simulink model "test2"  (R2020b)
settings: Solver=FixedStepAuto  StartTime=0.0  StopTime=10.0  RelTol=1e-3
model workspace (MAT data in the model file):
  HDLVAXIMasterConfig = hdlverifier.internal.AXIMaster.ConfigParams
libraries: hdlsllib x38
(part 1 of 2)
settings Model: Creator=horse  LastModifiedBy=horse
settings OptimizationCC: BlockReduction=off  ConditionallyExecuteInputs=off  DefaultParameterBehavior=Inlined  OptimizeBlockIOStorage=off
settings HardwareCC: TargetBitPerPointer=64  TargetBitPerSizeT=64  TargetBitPerPtrDiffT=64  TargetLongLongMode=on  TargetIntDivRoundTo=Zero  TargetEndianess=LittleEndian  TargetWordSize=64  TargetHWDeviceType=Generic->Custom  ProdEqTarget=off
settings RTWCC: Description=SystemVerilog DPI Component Generator  SystemTargetFile=systemverilog_dpi_grt.tlc  TemplateMakefile=systemverilog_dpi_grt_default_tmf
settings CodeAppCC: MaxIdLength=256
settings DPIGRTTargetCC: TargetFcnLib=ansi_tfl_table_tmw.mat  GenFloatMathFcnCalls=NOT IN USE  TargetLangStandard=C89/C90 (ANSI)  CodeReplacementLibrary=None  UtilityFuncGeneration=Auto  MultiwordTypeDef=System defined  MultiwordLength=2048  DynamicStringBufferSize=256  GenerateFullHeader=on  InferredTypesCompatibility=off  GenerateSampleERTMain=off  GenerateTestInterfaces=off  ModelReferenceCompliant=on  ParMdlRefBuildCompliant=on  CompOptLevelCompliant=off  ConcurrentExecutionCompliant=off  IncludeMdlTerminateFcn=on  CombineOutputUpdateFcns=off  CombineSignalStateStructs=on  GroupInternalDataByFunction=off  SuppressErrorStatus=off  IncludeFileDelimiter=Auto  ERTCustomFileBanners=off  SupportAbsoluteTime=on  LogVarNameModifier=rt_  MatFileLogging=off  CodeInterfacePackaging=Reusable function  PurelyIntegerCode=off  SupportNonFinite=on  SupportComplex=on  SupportContinuousTime=on  SupportNonInlinedSFcns=on  RemoveDisableFunc=off  RemoveResetFunc=off  SupportVariableSizeSignals=off  ParenthesesLevel=Nominal  CastingMode=Nominal  MATLABClassNameForMDSCustomization=Simulink.SoftwareTarget.TargetSpecificTriggerConfigurationBase  ModelStepFunctionPrototypeControlCompliant=off  CPPClassGenCompliant=off  AutosarCompliant=off  MDXCompliant=off  GRTInterface=off  GenerateAllocFcn=on  UseToolchainInfoCompliant=on  GenerateSharedConstants=on  CoderGroups=[]  AccessMethods=[]  LookupTableObjectStructAxisOrder=1,2,3,4,...  LUTObjectStructOrderExplicitValues=Size,Breakpoints,Table  LUTObjectStructOrderEvenSpacing=Size,Breakpoints,Table  ArrayLayout=Column-major  UnsupportedSFcnMsg=error  ERTHeaderFileRootName=$R$E  ERTSourceFileRootName=$R$E  ERTDataFileRootName=$R_data  RTWCAPISignals=on  RTWCAPIParams=off  RTWCAPIStates=off  RTWCAPIRootIO=off  ExtMode=off  ExtModeTransport=0  ExtModeStaticAlloc=off  ExtModeStaticAllocSize=1000000  ExtModeTesting=off  ExtModeMexFile=ext_comm  GenerateASAP2=off  MultiInstanceErrorCode=Error  DPICustomizeSystemVerilogCode=off  DPISystemVerilogTemplate=svdpi_event.vgt  DPIReportRunTimeError=off  DPIRunTimeErrorSeverity=Fatal  DPIGenerateTestBench=off  DPITestBenchSimulator=Mentor Graphics Questasim  DPITestPointAccessFcnInterface=None  DPIFixedPointDataType=CompatibleCType  DPIPortConnection=Port list  DPICompositeDataType=Flattened

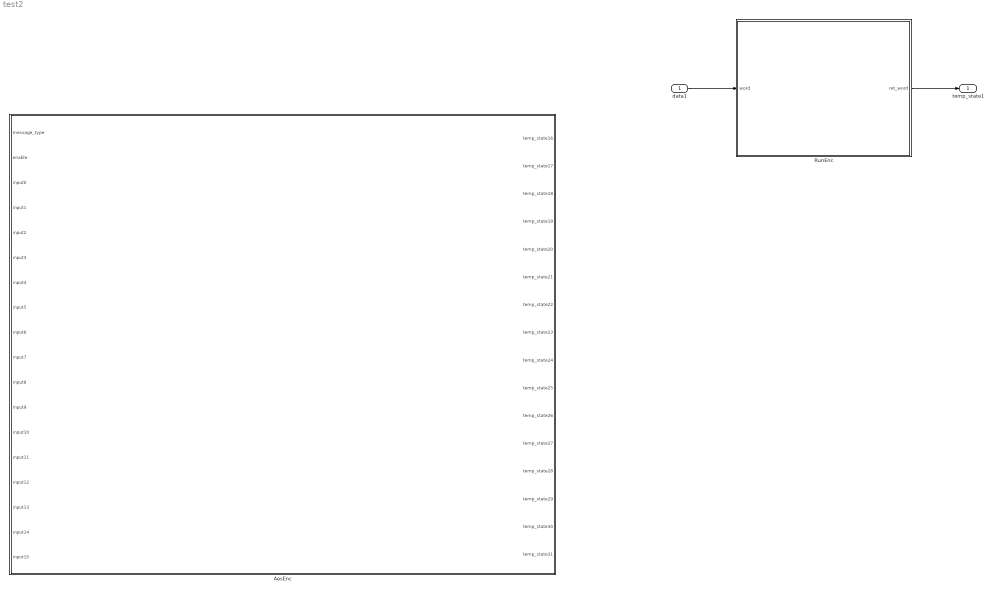
== system test2 ==
  data1 : Inport  OutDataTypeStr=uint32
  AesEnc : Subsystem
  RunEnc : MATLAB Function  TreatAsAtomicUnit=on
  temp_state1 : Outport  OutDataTypeStr=uint32  VectorParamsAs1DForOutWhenUnconnected=off
  wires:
  data1/1 -> RunEnc/1(word)
  RunEnc/1(ret_word) -> temp_state1/1

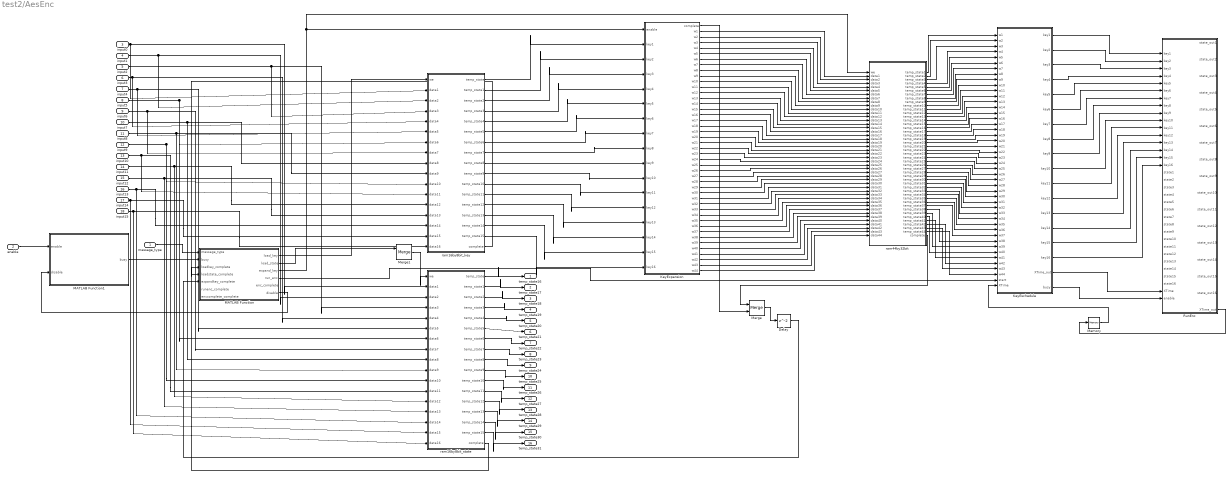
== system test2/AesEnc ==
  message_type : Inport  OutDataTypeStr=uint8
  enable : Inport  Port=2  OutDataTypeStr=boolean
  input0 : Inport  Port=3  OutDataTypeStr=uint8
  input1 : Inport  Port=4  OutDataTypeStr=uint8
  input2 : Inport  Port=5  OutDataTypeStr=uint8
  input3 : Inport  Port=6  OutDataTypeStr=uint8
  input4 : Inport  Port=7  OutDataTypeStr=uint8
  input5 : Inport  Port=8  OutDataTypeStr=uint8
  input6 : Inport  Port=9  OutDataTypeStr=uint8
  input7 : Inport  Port=10  OutDataTypeStr=uint8
  input8 : Inport  Port=11  OutDataTypeStr=uint8
  input9 : Inport  Port=12  OutDataTypeStr=uint8
  input10 : Inport  Port=13  OutDataTypeStr=uint8
  input11 : Inport  Port=14  OutDataTypeStr=uint8
  input12 : Inport  Port=15  OutDataTypeStr=uint8
  input13 : Inport  Port=16  OutDataTypeStr=uint8
  input14 : Inport  Port=17  OutDataTypeStr=uint8
  input15 : Inport  Port=18  OutDataTypeStr=uint8
  Delay : Delay  InitialCondition=0
  KeyEschedule : MATLAB Function  TreatAsAtomicUnit=on
  KeyExpansion : MATLAB Function  TreatAsAtomicUnit=on
  MATLAB Function : MATLAB Function  TreatAsAtomicUnit=on
  MATLAB Function1 : MATLAB Function  TreatAsAtomicUnit=on
  Memory : Memory  InheritSampleTime=on  LinearizeAsDelay=on
  Merge : Merge
  Merge1 : Merge
  RunEnc : MATLAB Function  TreatAsAtomicUnit=on
  ram16by8bit_key : Subsystem  TreatAsAtomicUnit=on
  ram16by8bit_state : Subsystem  TreatAsAtomicUnit=on
  ram44by32bit : Subsystem
  temp_state16 : Outport  OutDataTypeStr=uint8  VectorParamsAs1DForOutWhenUnconnected=off
  temp_state17 : Outport  Port=2  OutDataTypeStr=uint8  VectorParamsAs1DForOutWhenUnconnected=off
  temp_state18 : Outport  Port=3  OutDataTypeStr=uint8  VectorParamsAs1DForOutWhenUnconnected=off
  temp_state19 : Outport  Port=4  OutDataTypeStr=uint8  VectorParamsAs1DForOutWhenUnconnected=off
  temp_state20 : Outport  Port=5  OutDataTypeStr=uint8  VectorParamsAs1DForOutWhenUnconnected=off
  temp_state21 : Outport  Port=6  OutDataTypeStr=uint8  VectorParamsAs1DForOutWhenUnconnected=off
  temp_state22 : Outport  Port=7  OutDataTypeStr=uint8  VectorParamsAs1DForOutWhenUnconnected=off
  temp_state23 : Outport  Port=8  OutDataTypeStr=uint8  VectorParamsAs1DForOutWhenUnconnected=off
  temp_state24 : Outport  Port=9  OutDataTypeStr=uint8  VectorParamsAs1DForOutWhenUnconnected=off
  temp_state25 : Outport  Port=10  OutDataTypeStr=uint8  VectorParamsAs1DForOutWhenUnconnected=off
  temp_state26 : Outport  Port=11  OutDataTypeStr=uint8  VectorParamsAs1DForOutWhenUnconnected=off
  temp_state27 : Outport  Port=12  OutDataTypeStr=uint8  VectorParamsAs1DForOutWhenUnconnected=off
  temp_state28 : Outport  Port=13  OutDataTypeStr=uint8  VectorParamsAs1DForOutWhenUnconnected=off
  temp_state29 : Outport  Port=14  OutDataTypeStr=uint8  VectorParamsAs1DForOutWhenUnconnected=off
  temp_state30 : Outport  Port=15  OutDataTypeStr=uint8  VectorParamsAs1DForOutWhenUnconnected=off
  temp_state31 : Outport  Port=16  OutDataTypeStr=uint8  VectorParamsAs1DForOutWhenUnconnected=off
  wires:
  MATLAB Function/6(disable) -> MATLAB Function1/2(disable)
  MATLAB Function1/1(busy) -> MATLAB Function/2(busy)
  message_type/1 -> MATLAB Function/1(message_type)
  MATLAB Function/1(load_key) -> ram16by8bit_key/1(we)
  ram16by8bit_state/15(temp_state14) -> temp_state30/1
  ram16by8bit_state/7(temp_state6) -> temp_state22/1
  ram16by8bit_state/2(temp_state1) -> temp_state17/1
  ram16by8bit_state/9(temp_state8) -> temp_state24/1
  ram16by8bit_state/5(temp_state4) -> temp_state20/1
  ram16by8bit_state/14(temp_state13) -> temp_state29/1
  ram16by8bit_state/12(temp_state11) -> temp_state27/1
  ram16by8bit_state/13(temp_state12) -> temp_state28/1
  ram16by8bit_state/4(temp_state3) -> temp_state19/1
  ram16by8bit_state/8(temp_state7) -> temp_state23/1
  ram16by8bit_state/1(temp_state) -> temp_state16/1
  ram16by8bit_state/10(temp_state9) -> temp_state25/1
  ram16by8bit_state/11(temp_state10) -> temp_state26/1
  ram16by8bit_state/16(temp_state15) -> temp_state31/1
  ram16by8bit_state/6(temp_state5) -> temp_state21/1
  ram16by8bit_state/3(temp_state2) -> temp_state18/1
  MATLAB Function/2(load_state) -> Merge1/1
  ram16by8bit_key/17(complete) -> MATLAB Function/3(loadkey_complete)
  ram16by8bit_state/17(complete) -> MATLAB Function/4(loadstate_complete)
  enable/1 -> MATLAB Function1/1(enable)
  KeyExpansion/1(complete) -> Merge/2
  Delay/1 -> MATLAB Function/5(expandkey_complete)
  input13/1 -> ram16by8bit_state/15(data14), ram16by8bit_key/15(data14)
  input9/1 -> ram16by8bit_state/11(data10), ram16by8bit_key/11(data10)
  input1/1 -> ram16by8bit_state/3(data2), ram16by8bit_key/3(data2)
  input15/1 -> ram16by8bit_state/17(data16), ram16by8bit_key/17(data16)
  input7/1 -> ram16by8bit_state/9(data8), ram16by8bit_key/9(data8)
  input3/1 -> ram16by8bit_state/5(data4), ram16by8bit_key/5(data4)
  input8/1 -> ram16by8bit_state/10(data9), ram16by8bit_key/10(data9)
  input5/1 -> ram16by8bit_state/7(data6), ram16by8bit_key/7(data6)
  input2/1 -> ram16by8bit_state/4(data3), ram16by8bit_key/4(data3)
  input4/1 -> ram16by8bit_state/6(data5), ram16by8bit_key/6(data5)
  input6/1 -> ram16by8bit_state/8(data7), ram16by8bit_key/8(data7)
  input14/1 -> ram16by8bit_state/16(data15), ram16by8bit_key/16(data15)
  input10/1 -> ram16by8bit_state/12(data11), ram16by8bit_key/12(data11)
  input11/1 -> ram16by8bit_state/13(data12), ram16by8bit_key/13(data12)
  input12/1 -> ram16by8bit_state/14(data13), ram16by8bit_key/14(data13)
  input0/1 -> ram16by8bit_state/2(data1), ram16by8bit_key/2(data1)
  MATLAB Function/3(expand_key) -> ram44by32bit/1(we), KeyExpansion/1(enable)
  ram16by8bit_key/1(temp_state) -> KeyExpansion/2(key1)
  ram16by8bit_key/2(temp_state1) -> KeyExpansion/3(key2)
  ram16by8bit_key/3(temp_state2) -> KeyExpansion/4(key3)
  ram16by8bit_key/4(temp_state3) -> KeyExpansion/5(key4)
  ram16by8bit_key/5(temp_state4) -> KeyExpansion/6(key5)
  ram16by8bit_key/6(temp_state5) -> KeyExpansion/7(key6)
  ram16by8bit_key/7(temp_state6) -> KeyExpansion/8(key7)
  ram16by8bit_key/8(temp_state7) -> KeyExpansion/9(key8)
  ram16by8bit_key/9(temp_state8) -> KeyExpansion/10(key9)
  ram16by8bit_key/10(temp_state9) -> KeyExpansion/11(key10)
  ram16by8bit_key/11(temp_state10) -> KeyExpansion/12(key11)
  ram16by8bit_key/12(temp_state11) -> KeyExpansion/13(key12)
  ram16by8bit_key/13(temp_state12) -> KeyExpansion/14(key13)
  ram16by8bit_key/14(temp_state13) -> KeyExpansion/15(key14)
  ram16by8bit_key/16(temp_state15) -> KeyExpansion/17(key16)
  ram16by8bit_key/15(temp_state14) -> KeyExpansion/16(key15)
  KeyExpansion/45(w44) -> ram44by32bit/45(data44)
  KeyExpansion/44(w43) -> ram44by32bit/44(data43)
  KeyExpansion/43(w42) -> ram44by32bit/43(data42)
  KeyExpansion/42(w41) -> ram44by32bit/42(data41)
  KeyExpansion/41(w40) -> ram44by32bit/41(data40)
  KeyExpansion/40(w39) -> ram44by32bit/40(data39)
  KeyExpansion/39(w38) -> ram44by32bit/39(data38)
  KeyExpansion/38(w37) -> ram44by32bit/38(data37)
  KeyExpansion/37(w36) -> ram44by32bit/37(data36)
  KeyExpansion/36(w35) -> ram44by32bit/36(data35)
  KeyExpansion/35(w34) -> ram44by32bit/35(data34)
  KeyExpansion/34(w33) -> ram44by32bit/34(data33)
  KeyExpansion/33(w32) -> ram44by32bit/33(data32)
  KeyExpansion/32(w31) -> ram44by32bit/32(data31)
  KeyExpansion/31(w30) -> ram44by32bit/31(data30)
  KeyExpansion/30(w29) -> ram44by32bit/30(data29)
  KeyExpansion/29(w28) -> ram44by32bit/29(data28)
  KeyExpansion/28(w27) -> ram44by32bit/28(data27)
  KeyExpansion/27(w26) -> ram44by32bit/27(data26)
  KeyExpansion/26(w25) -> ram44by32bit/26(data25)
  KeyExpansion/25(w24) -> ram44by32bit/25(data24)
  KeyExpansion/24(w23) -> ram44by32bit/24(data23)
  KeyExpansion/23(w22) -> ram44by32bit/23(data22)
  KeyExpansion/22(w21) -> ram44by32bit/22(data21)
  KeyExpansion/21(w20) -> ram44by32bit/21(data20)
  KeyExpansion/20(w19) -> ram44by32bit/20(data19)
  KeyExpansion/19(w18) -> ram44by32bit/19(data18)
  KeyExpansion/18(w17) -> ram44by32bit/18(data17)
  KeyExpansion/17(w16) -> ram44by32bit/17(data16)
  KeyExpansion/16(w15) -> ram44by32bit/16(data15)
  KeyExpansion/15(w14) -> ram44by32bit/15(data14)
  KeyExpansion/14(w13) -> ram44by32bit/14(data13)
  KeyExpansion/13(w12) -> ram44by32bit/13(data12)
  KeyExpansion/12(w11) -> ram44by32bit/12(data11)
  KeyExpansion/11(w10) -> ram44by32bit/11(data10)
  KeyExpansion/10(w9) -> ram44by32bit/10(data9)
  KeyExpansion/9(w8) -> ram44by32bit/9(data8)
  KeyExpansion/8(w7) -> ram44by32bit/8(data7)
  KeyExpansion/7(w6) -> ram44by32bit/7(data6)
  KeyExpansion/6(w5) -> ram44by32bit/6(data5)
  KeyExpansion/5(w4) -> ram44by32bit/5(data4)
  KeyExpansion/4(w3) -> ram44by32bit/4(data3)
  KeyExpansion/3(w2) -> ram44by32bit/3(data2)
  KeyExpansion/2(w1) -> ram44by32bit/2(data1)
  ram44by32bit/45(complete) -> Merge/1
  Merge/1 -> Delay/1
  KeyEschedule/17(XTime_out) -> RunEnc/33(XTime)
  Memory/1 -> KeyEschedule/46(XTime)
  ram44by32bit/1(temp_state1) -> KeyEschedule/1(w1)
  ram44by32bit/2(temp_state2) -> KeyEschedule/2(w2)
  ram44by32bit/3(temp_state3) -> KeyEschedule/3(w3)
  ram44by32bit/4(temp_state4) -> KeyEschedule/4(w4)
  ram44by32bit/5(temp_state5) -> KeyEschedule/5(w5)
  ram44by32bit/6(temp_state6) -> KeyEschedule/6(w6)
  ram44by32bit/7(temp_state7) -> KeyEschedule/7(w7)
  ram44by32bit/8(temp_state8) -> KeyEschedule/8(w8)
  ram44by32bit/9(temp_state9) -> KeyEschedule/9(w9)
  ram44by32bit/10(temp_state10) -> KeyEschedule/10(w10)
  ram44by32bit/11(temp_state11) -> KeyEschedule/11(w11)
  ram44by32bit/12(temp_state12) -> KeyEschedule/12(w12)
  ram44by32bit/13(temp_state13) -> KeyEschedule/13(w13)
  ram44by32bit/14(temp_state14) -> KeyEschedule/14(w14)
  ram44by32bit/15(temp_state15) -> KeyEschedule/15(w15)
  ram44by32bit/16(temp_state16) -> KeyEschedule/16(w16)
  ram44by32bit/17(temp_state17) -> KeyEschedule/17(w17)
  ram44by32bit/18(temp_state18) -> KeyEschedule/18(w18)
  ram44by32bit/19(temp_state19) -> KeyEschedule/19(w19)
  ram44by32bit/20(temp_state20) -> KeyEschedule/20(w20)
  ram44by32bit/21(temp_state21) -> KeyEschedule/21(w21)
  ram44by32bit/22(temp_state22) -> KeyEschedule/22(w22)
  ram44by32bit/23(temp_state23) -> KeyEschedule/23(w23)
  ram44by32bit/24(temp_state24) -> KeyEschedule/24(w24)
  ram44by32bit/25(temp_state25) -> KeyEschedule/25(w25)
  ram44by32bit/26(temp_state26) -> KeyEschedule/26(w26)
  ram44by32bit/27(temp_state27) -> KeyEschedule/27(w27)
  ram44by32bit/28(temp_state28) -> KeyEschedule/28(w28)
  ram44by32bit/29(temp_state29) -> KeyEschedule/29(w29)
  ram44by32bit/30(temp_state30) -> KeyEschedule/30(w30)
  ram44by32bit/31(temp_state31) -> KeyEschedule/31(w31)
  ram44by32bit/32(temp_state32) -> KeyEschedule/32(w32)
  ram44by32bit/33(temp_state33) -> KeyEschedule/33(w33)
  ram44by32bit/34(temp_state34) -> KeyEschedule/34(w34)
  ram44by32bit/35(temp_state35) -> KeyEschedule/35(w35)
  ram44by32bit/36(temp_state36) -> KeyEschedule/36(w36)
  ram44by32bit/37(temp_state37) -> KeyEschedule/37(w37)
  ram44by32bit/38(temp_state38) -> KeyEschedule/38(w38)
  ram44by32bit/39(temp_state39) -> KeyEschedule/39(w39)
  ram44by32bit/40(temp_state40) -> KeyEschedule/40(w40)
  ram44by32bit/41(temp_state41) -> KeyEschedule/41(w41)
  ram44by32bit/42(temp_state42) -> KeyEschedule/42(w42)
  ram44by32bit/43(temp_state43) -> KeyEschedule/43(w43)
  ram44by32bit/44(temp_state44) -> KeyEschedule/44(w44)
  MATLAB Function/4(run_enc) -> KeyEschedule/45(start)
  RunEnc/17(XTime_out) -> Memory/1
  KeyEschedule/18(busy) -> RunEnc/34(enable)
  Merge1/1 -> ram16by8bit_state/1(we)
  KeyEschedule/1(key1) -> RunEnc/1(key1)
  KeyEschedule/2(key2) -> RunEnc/2(key2)
  KeyEschedule/3(key3) -> RunEnc/3(key3)
  KeyEschedule/4(key4) -> RunEnc/4(key4)
  KeyEschedule/5(key5) -> RunEnc/5(key5)
  KeyEschedule/6(key6) -> RunEnc/6(key6)
  KeyEschedule/7(key7) -> RunEnc/7(key7)
  KeyEschedule/8(key8) -> RunEnc/8(key8)
  KeyEschedule/9(key9) -> RunEnc/9(key9)
  KeyEschedule/10(key10) -> RunEnc/10(key10)
  KeyEschedule/11(key11) -> RunEnc/11(key11)
  KeyEschedule/12(key12) -> RunEnc/12(key12)
  KeyEschedule/13(key13) -> RunEnc/13(key13)
  KeyEschedule/14(key14) -> RunEnc/14(key14)
  KeyEschedule/15(key15) -> RunEnc/15(key15)
  KeyEschedule/16(key16) -> RunEnc/16(key16)

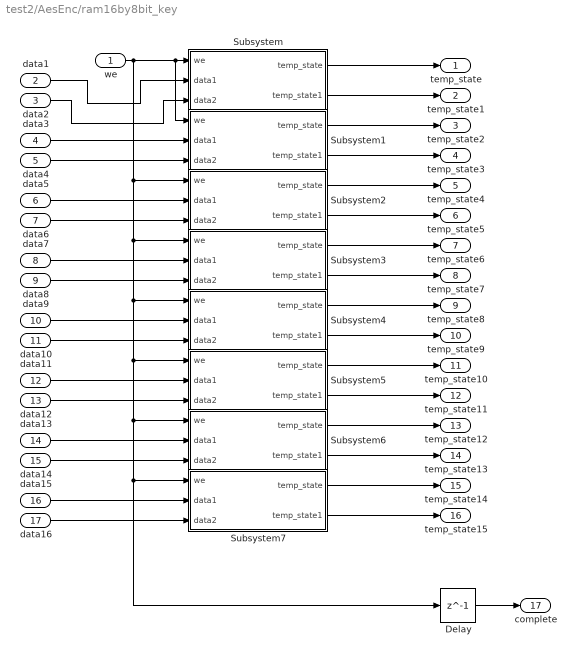
== system test2/AesEnc/ram16by8bit_key ==
  we : Inport  OutDataTypeStr=boolean
  data1 : Inport  Port=2  OutDataTypeStr=uint8
  data2 : Inport  Port=3  OutDataTypeStr=uint8
  data3 : Inport  Port=4  OutDataTypeStr=uint8
  data4 : Inport  Port=5  OutDataTypeStr=uint8
  data5 : Inport  Port=6  OutDataTypeStr=uint8
  data6 : Inport  Port=7  OutDataTypeStr=uint8
  data7 : Inport  Port=8  OutDataTypeStr=uint8
  data8 : Inport  Port=9  OutDataTypeStr=uint8
  data9 : Inport  Port=10  OutDataTypeStr=uint8
  data10 : Inport  Port=11  OutDataTypeStr=uint8
  data11 : Inport  Port=12  OutDataTypeStr=uint8
  data12 : Inport  Port=13  OutDataTypeStr=uint8
  data13 : Inport  Port=14  OutDataTypeStr=uint8
  data14 : Inport  Port=15  OutDataTypeStr=uint8
  data15 : Inport  Port=16  OutDataTypeStr=uint8
  data16 : Inport  Port=17  OutDataTypeStr=uint8
  Delay : Delay  DelayLength=1  InitialCondition=0
  Subsystem : Subsystem
  Subsystem1 : Subsystem
  Subsystem2 : Subsystem
  Subsystem3 : Subsystem
  Subsystem4 : Subsystem
  Subsystem5 : Subsystem
  Subsystem6 : Subsystem
  Subsystem7 : Subsystem
  temp_state : Outport  OutDataTypeStr=uint8  VectorParamsAs1DForOutWhenUnconnected=off
  temp_state1 : Outport  Port=2  OutDataTypeStr=uint8  VectorParamsAs1DForOutWhenUnconnected=off
  temp_state2 : Outport  Port=3  OutDataTypeStr=uint8  VectorParamsAs1DForOutWhenUnconnected=off
  temp_state3 : Outport  Port=4  OutDataTypeStr=uint8  VectorParamsAs1DForOutWhenUnconnected=off
  temp_state4 : Outport  Port=5  OutDataTypeStr=uint8  VectorParamsAs1DForOutWhenUnconnected=off
  temp_state5 : Outport  Port=6  OutDataTypeStr=uint8  VectorParamsAs1DForOutWhenUnconnected=off
  temp_state6 : Outport  Port=7  OutDataTypeStr=uint8  VectorParamsAs1DForOutWhenUnconnected=off
  temp_state7 : Outport  Port=8  OutDataTypeStr=uint8  VectorParamsAs1DForOutWhenUnconnected=off
  temp_state8 : Outport  Port=9  OutDataTypeStr=uint8  VectorParamsAs1DForOutWhenUnconnected=off
  temp_state9 : Outport  Port=10  OutDataTypeStr=uint8  VectorParamsAs1DForOutWhenUnconnected=off
  temp_state10 : Outport  Port=11  OutDataTypeStr=uint8  VectorParamsAs1DForOutWhenUnconnected=off
  temp_state11 : Outport  Port=12  OutDataTypeStr=uint8  VectorParamsAs1DForOutWhenUnconnected=off
  temp_state12 : Outport  Port=13  OutDataTypeStr=uint8  VectorParamsAs1DForOutWhenUnconnected=off
  temp_state13 : Outport  Port=14  OutDataTypeStr=uint8  VectorParamsAs1DForOutWhenUnconnected=off
  temp_state14 : Outport  Port=15  OutDataTypeStr=uint8  VectorParamsAs1DForOutWhenUnconnected=off
  temp_state15 : Outport  Port=16  OutDataTypeStr=uint8  VectorParamsAs1DForOutWhenUnconnected=off
  complete : Outport  Port=17  OutDataTypeStr=boolean  VectorParamsAs1DForOutWhenUnconnected=off
  wires:
  Subsystem1/1(temp_state) -> temp_state2/1
  Subsystem5/1(temp_state) -> temp_state10/1
  data4/1 -> Subsystem1/3(data2)
  data15/1 -> Subsystem7/2(data1)
  data6/1 -> Subsystem2/3(data2)
  Subsystem/2(temp_state1) -> temp_state1/1
  data2/1 -> Subsystem/3(data2)
  data1/1 -> Subsystem/2(data1)
  data10/1 -> Subsystem4/3(data2)
  Subsystem1/2(temp_state1) -> temp_state3/1
  Subsystem/1(temp_state) -> temp_state/1
  data11/1 -> Subsystem5/2(data1)
  Subsystem6/1(temp_state) -> temp_state12/1
  Subsystem2/1(temp_state) -> temp_state4/1
  data16/1 -> Subsystem7/3(data2)
  Subsystem2/2(temp_state1) -> temp_state5/1
  data5/1 -> Subsystem2/2(data1)
  data3/1 -> Subsystem1/2(data1)
  data12/1 -> Subsystem5/3(data2)
  Subsystem3/1(temp_state) -> temp_state6/1
  data14/1 -> Subsystem6/3(data2)
  Subsystem3/2(temp_state1) -> temp_state7/1
  data8/1 -> Subsystem3/3(data2)
  data9/1 -> Subsystem4/2(data1)
  Subsystem7/1(temp_state) -> temp_state14/1
  data7/1 -> Subsystem3/2(data1)
  Subsystem5/2(temp_state1) -> temp_state11/1
  data13/1 -> Subsystem6/2(data1)
  Subsystem7/2(temp_state1) -> temp_state15/1
  Subsystem6/2(temp_state1) -> temp_state13/1
  Subsystem4/1(temp_state) -> temp_state8/1
  Subsystem4/2(temp_state1) -> temp_state9/1
  we/1 -> Delay/1, Subsystem7/1(we), Subsystem6/1(we), Subsystem5/1(we), Subsystem4/1(we), Subsystem3/1(we), Subsystem2/1(we), Subsystem1/1(we), Subsystem/1(we)
  Delay/1 -> complete/1

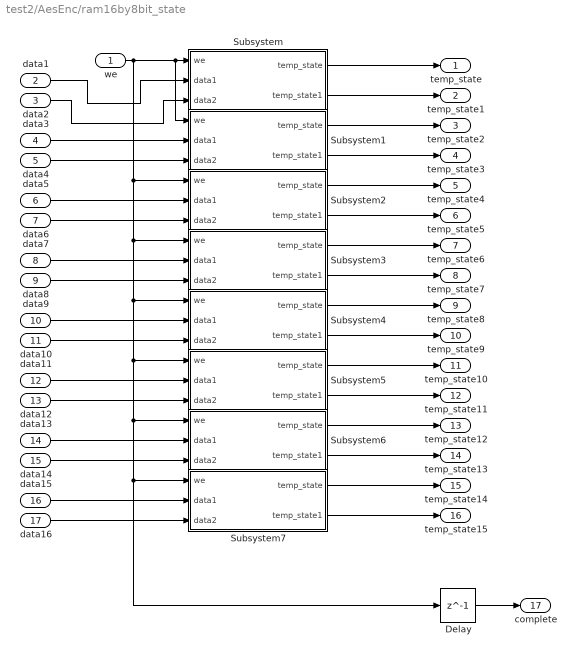
== system test2/AesEnc/ram16by8bit_state ==
  we : Inport  OutDataTypeStr=boolean
  data1 : Inport  Port=2  OutDataTypeStr=uint8
  data2 : Inport  Port=3  OutDataTypeStr=uint8
  data3 : Inport  Port=4  OutDataTypeStr=uint8
  data4 : Inport  Port=5  OutDataTypeStr=uint8
  data5 : Inport  Port=6  OutDataTypeStr=uint8
  data6 : Inport  Port=7  OutDataTypeStr=uint8
  data7 : Inport  Port=8  OutDataTypeStr=uint8
  data8 : Inport  Port=9  OutDataTypeStr=uint8
  data9 : Inport  Port=10  OutDataTypeStr=uint8
  data10 : Inport  Port=11  OutDataTypeStr=uint8
  data11 : Inport  Port=12  OutDataTypeStr=uint8
  data12 : Inport  Port=13  OutDataTypeStr=uint8
  data13 : Inport  Port=14  OutDataTypeStr=uint8
  data14 : Inport  Port=15  OutDataTypeStr=uint8
  data15 : Inport  Port=16  OutDataTypeStr=uint8
  data16 : Inport  Port=17  OutDataTypeStr=uint8
  Delay : Delay  DelayLength=1  InitialCondition=0
  Subsystem : Subsystem
  Subsystem1 : Subsystem
  Subsystem2 : Subsystem
  Subsystem3 : Subsystem
  Subsystem4 : Subsystem
  Subsystem5 : Subsystem
  Subsystem6 : Subsystem
  Subsystem7 : Subsystem
  temp_state : Outport  OutDataTypeStr=uint8  VectorParamsAs1DForOutWhenUnconnected=off
  temp_state1 : Outport  Port=2  OutDataTypeStr=uint8  VectorParamsAs1DForOutWhenUnconnected=off
  temp_state2 : Outport  Port=3  OutDataTypeStr=uint8  VectorParamsAs1DForOutWhenUnconnected=off
  temp_state3 : Outport  Port=4  OutDataTypeStr=uint8  VectorParamsAs1DForOutWhenUnconnected=off
  temp_state4 : Outport  Port=5  OutDataTypeStr=uint8  VectorParamsAs1DForOutWhenUnconnected=off
  temp_state5 : Outport  Port=6  OutDataTypeStr=uint8  VectorParamsAs1DForOutWhenUnconnected=off
  temp_state6 : Outport  Port=7  OutDataTypeStr=uint8  VectorParamsAs1DForOutWhenUnconnected=off
  temp_state7 : Outport  Port=8  OutDataTypeStr=uint8  VectorParamsAs1DForOutWhenUnconnected=off
  temp_state8 : Outport  Port=9  OutDataTypeStr=uint8  VectorParamsAs1DForOutWhenUnconnected=off
  temp_state9 : Outport  Port=10  OutDataTypeStr=uint8  VectorParamsAs1DForOutWhenUnconnected=off
  temp_state10 : Outport  Port=11  OutDataTypeStr=uint8  VectorParamsAs1DForOutWhenUnconnected=off
  temp_state11 : Outport  Port=12  OutDataTypeStr=uint8  VectorParamsAs1DForOutWhenUnconnected=off
  temp_state12 : Outport  Port=13  OutDataTypeStr=uint8  VectorParamsAs1DForOutWhenUnconnected=off
  temp_state13 : Outport  Port=14  OutDataTypeStr=uint8  VectorParamsAs1DForOutWhenUnconnected=off
  temp_state14 : Outport  Port=15  OutDataTypeStr=uint8  VectorParamsAs1DForOutWhenUnconnected=off
  temp_state15 : Outport  Port=16  OutDataTypeStr=uint8  VectorParamsAs1DForOutWhenUnconnected=off
  complete : Outport  Port=17  OutDataTypeStr=boolean  VectorParamsAs1DForOutWhenUnconnected=off
  wires:
  Subsystem1/1(temp_state) -> temp_state2/1
  Subsystem5/1(temp_state) -> temp_state10/1
  data4/1 -> Subsystem1/3(data2)
  data15/1 -> Subsystem7/2(data1)
  data6/1 -> Subsystem2/3(data2)
  Subsystem/2(temp_state1) -> temp_state1/1
  data2/1 -> Subsystem/3(data2)
  data1/1 -> Subsystem/2(data1)
  data10/1 -> Subsystem4/3(data2)
  Subsystem1/2(temp_state1) -> temp_state3/1
  Subsystem/1(temp_state) -> temp_state/1
  data11/1 -> Subsystem5/2(data1)
  Subsystem6/1(temp_state) -> temp_state12/1
  Subsystem2/1(temp_state) -> temp_state4/1
  data16/1 -> Subsystem7/3(data2)
  Subsystem2/2(temp_state1) -> temp_state5/1
  data5/1 -> Subsystem2/2(data1)
  data3/1 -> Subsystem1/2(data1)
  data12/1 -> Subsystem5/3(data2)
  Subsystem3/1(temp_state) -> temp_state6/1
  data14/1 -> Subsystem6/3(data2)
  Subsystem3/2(temp_state1) -> temp_state7/1
  data8/1 -> Subsystem3/3(data2)
  data9/1 -> Subsystem4/2(data1)
  Subsystem7/1(temp_state) -> temp_state14/1
  data7/1 -> Subsystem3/2(data1)
  Subsystem5/2(temp_state1) -> temp_state11/1
  data13/1 -> Subsystem6/2(data1)
  Subsystem7/2(temp_state1) -> temp_state15/1
  Subsystem6/2(temp_state1) -> temp_state13/1
  Subsystem4/1(temp_state) -> temp_state8/1
  Subsystem4/2(temp_state1) -> temp_state9/1
  we/1 -> Delay/1, Subsystem7/1(we), Subsystem6/1(we), Subsystem5/1(we), Subsystem4/1(we), Subsystem3/1(we), Subsystem2/1(we), Subsystem1/1(we), Subsystem/1(we)
  Delay/1 -> complete/1

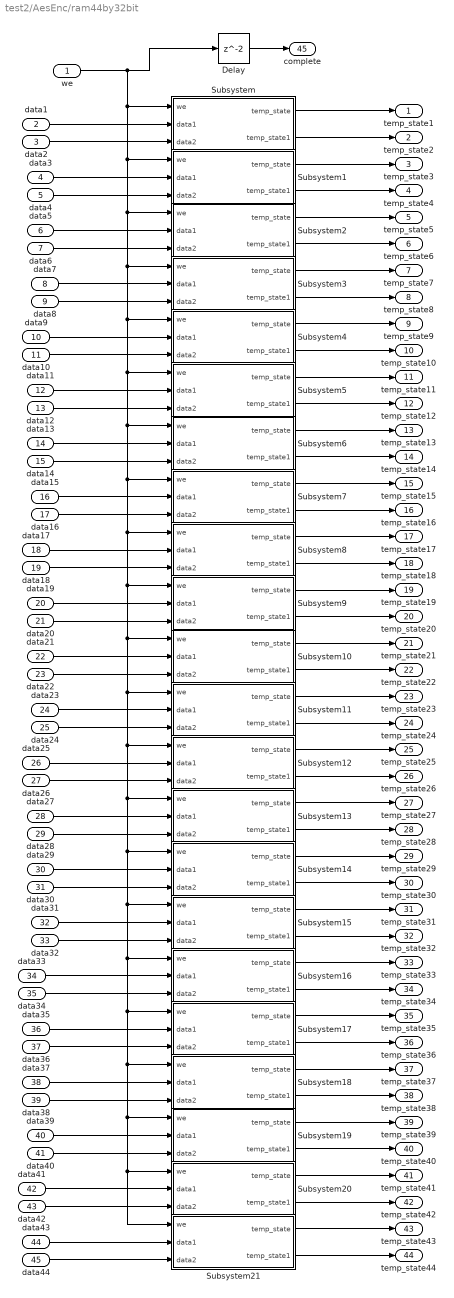
== system test2/AesEnc/ram44by32bit ==
  we : Inport  OutDataTypeStr=boolean
  data1 : Inport  Port=2  OutDataTypeStr=uint32
  data2 : Inport  Port=3  OutDataTypeStr=uint32
  data3 : Inport  Port=4  OutDataTypeStr=uint32
  data4 : Inport  Port=5  OutDataTypeStr=uint32
  data5 : Inport  Port=6  OutDataTypeStr=uint32
  data6 : Inport  Port=7  OutDataTypeStr=uint32
  data7 : Inport  Port=8  OutDataTypeStr=uint32
  data8 : Inport  Port=9  OutDataTypeStr=uint32
  data9 : Inport  Port=10  OutDataTypeStr=uint32
  data10 : Inport  Port=11  OutDataTypeStr=uint32
  data11 : Inport  Port=12  OutDataTypeStr=uint32
  data12 : Inport  Port=13  OutDataTypeStr=uint32
  data13 : Inport  Port=14  OutDataTypeStr=uint32
  data14 : Inport  Port=15  OutDataTypeStr=uint32
  data15 : Inport  Port=16  OutDataTypeStr=uint32
  data16 : Inport  Port=17  OutDataTypeStr=uint32
  data17 : Inport  Port=18  OutDataTypeStr=uint32
  data18 : Inport  Port=19  OutDataTypeStr=uint32
  data19 : Inport  Port=20  OutDataTypeStr=uint32
  data20 : Inport  Port=21  OutDataTypeStr=uint32
  data21 : Inport  Port=22  OutDataTypeStr=uint32
  data22 : Inport  Port=23  OutDataTypeStr=uint32
  data23 : Inport  Port=24  OutDataTypeStr=uint32
  data24 : Inport  Port=25  OutDataTypeStr=uint32
  data25 : Inport  Port=26  OutDataTypeStr=uint32
  data26 : Inport  Port=27  OutDataTypeStr=uint32
  data27 : Inport  Port=28  OutDataTypeStr=uint32
  data28 : Inport  Port=29  OutDataTypeStr=uint32
  data29 : Inport  Port=30  OutDataTypeStr=uint32
  data30 : Inport  Port=31  OutDataTypeStr=uint32
  data31 : Inport  Port=32  OutDataTypeStr=uint32
  data32 : Inport  Port=33  OutDataTypeStr=uint32
  data33 : Inport  Port=34  OutDataTypeStr=uint32
  data34 : Inport  Port=35  OutDataTypeStr=uint32
  data35 : Inport  Port=36  OutDataTypeStr=uint32
  data36 : Inport  Port=37  OutDataTypeStr=uint32
  data37 : Inport  Port=38  OutDataTypeStr=uint32
  data38 : Inport  Port=39  OutDataTypeStr=uint32
  data39 : Inport  Port=40  OutDataTypeStr=uint32
  data40 : Inport  Port=41  OutDataTypeStr=uint32
  data41 : Inport  Port=42  OutDataTypeStr=uint32
  data42 : Inport  Port=43  OutDataTypeStr=uint32
  data43 : Inport  Port=44  OutDataTypeStr=uint32
  data44 : Inport  Port=45  OutDataTypeStr=uint32
  Delay : Delay  InitialCondition=0
  Subsystem : Subsystem
  Subsystem1 : Subsystem
  Subsystem10 : Subsystem
  Subsystem11 : Subsystem
  Subsystem12 : Subsystem
  Subsystem13 : Subsystem
  Subsystem14 : Subsystem
  Subsystem15 : Subsystem
  Subsystem16 : Subsystem
  Subsystem17 : Subsystem
  Subsystem18 : Subsystem
  Subsystem19 : Subsystem
  Subsystem2 : Subsystem
  Subsystem20 : Subsystem
  Subsystem21 : Subsystem
  Subsystem3 : Subsystem
  Subsystem4 : Subsystem
  Subsystem5 : Subsystem
  Subsystem6 : Subsystem
  Subsystem7 : Subsystem
  Subsystem8 : Subsystem
  Subsystem9 : Subsystem
  temp_state1 : Outport  OutDataTypeStr=uint32  VectorParamsAs1DForOutWhenUnconnected=off
  temp_state2 : Outport  Port=2  OutDataTypeStr=uint32  VectorParamsAs1DForOutWhenUnconnected=off
  temp_state3 : Outport  Port=3  OutDataTypeStr=uint32  VectorParamsAs1DForOutWhenUnconnected=off
  temp_state4 : Outport  Port=4  OutDataTypeStr=uint32  VectorParamsAs1DForOutWhenUnconnected=off
  temp_state5 : Outport  Port=5  OutDataTypeStr=uint32  VectorParamsAs1DForOutWhenUnconnected=off
  temp_state6 : Outport  Port=6  OutDataTypeStr=uint32  VectorParamsAs1DForOutWhenUnconnected=off
  temp_state7 : Outport  Port=7  OutDataTypeStr=uint32  VectorParamsAs1DForOutWhenUnconnected=off
  temp_state8 : Outport  Port=8  OutDataTypeStr=uint32  VectorParamsAs1DForOutWhenUnconnected=off
  temp_state9 : Outport  Port=9  OutDataTypeStr=uint32  VectorParamsAs1DForOutWhenUnconnected=off
  temp_state10 : Outport  Port=10  OutDataTypeStr=uint32  VectorParamsAs1DForOutWhenUnconnected=off
  temp_state11 : Outport  Port=11  OutDataTypeStr=uint32  VectorParamsAs1DForOutWhenUnconnected=off
  temp_state12 : Outport  Port=12  OutDataTypeStr=uint32  VectorParamsAs1DForOutWhenUnconnected=off
  temp_state13 : Outport  Port=13  OutDataTypeStr=uint32  VectorParamsAs1DForOutWhenUnconnected=off
  temp_state14 : Outport  Port=14  OutDataTypeStr=uint32  VectorParamsAs1DForOutWhenUnconnected=off
  temp_state15 : Outport  Port=15  OutDataTypeStr=uint32  VectorParamsAs1DForOutWhenUnconnected=off
  temp_state16 : Outport  Port=16  OutDataTypeStr=uint32  VectorParamsAs1DForOutWhenUnconnected=off
  temp_state17 : Outport  Port=17  OutDataTypeStr=uint32  VectorParamsAs1DForOutWhenUnconnected=off
  temp_state18 : Outport  Port=18  OutDataTypeStr=uint32  VectorParamsAs1DForOutWhenUnconnected=off
  temp_state19 : Outport  Port=19  OutDataTypeStr=uint32  VectorParamsAs1DForOutWhenUnconnected=off
  temp_state20 : Outport  Port=20  OutDataTypeStr=uint32  VectorParamsAs1DForOutWhenUnconnected=off
  temp_state21 : Outport  Port=21  OutDataTypeStr=uint32  VectorParamsAs1DForOutWhenUnconnected=off
  temp_state22 : Outport  Port=22  OutDataTypeStr=uint32  VectorParamsAs1DForOutWhenUnconnected=off
  temp_state23 : Outport  Port=23  OutDataTypeStr=uint32  VectorParamsAs1DForOutWhenUnconnected=off
  temp_state24 : Outport  Port=24  OutDataTypeStr=uint32  VectorParamsAs1DForOutWhenUnconnected=off
  temp_state25 : Outport  Port=25  OutDataTypeStr=uint32  VectorParamsAs1DForOutWhenUnconnected=off
  temp_state26 : Outport  Port=26  OutDataTypeStr=uint32  VectorParamsAs1DForOutWhenUnconnected=off
  temp_state27 : Outport  Port=27  OutDataTypeStr=uint32  VectorParamsAs1DForOutWhenUnconnected=off
  temp_state28 : Outport  Port=28  OutDataTypeStr=uint32  VectorParamsAs1DForOutWhenUnconnected=off
  temp_state29 : Outport  Port=29  OutDataTypeStr=uint32  VectorParamsAs1DForOutWhenUnconnected=off
  temp_state30 : Outport  Port=30  OutDataTypeStr=uint32  VectorParamsAs1DForOutWhenUnconnected=off
  temp_state31 : Outport  Port=31  OutDataTypeStr=uint32  VectorParamsAs1DForOutWhenUnconnected=off
  temp_state32 : Outport  Port=32  OutDataTypeStr=uint32  VectorParamsAs1DForOutWhenUnconnected=off
  temp_state33 : Outport  Port=33  OutDataTypeStr=uint32  VectorParamsAs1DForOutWhenUnconnected=off
  temp_state34 : Outport  Port=34  OutDataTypeStr=uint32  VectorParamsAs1DForOutWhenUnconnected=off
  temp_state35 : Outport  Port=35  OutDataTypeStr=uint32  VectorParamsAs1DForOutWhenUnconnected=off
  temp_state36 : Outport  Port=36  OutDataTypeStr=uint32  VectorParamsAs1DForOutWhenUnconnected=off
  temp_state37 : Outport  Port=37  OutDataTypeStr=uint32  VectorParamsAs1DForOutWhenUnconnected=off
  temp_state38 : Outport  Port=38  OutDataTypeStr=uint32  VectorParamsAs1DForOutWhenUnconnected=off
  temp_state39 : Outport  Port=39  OutDataTypeStr=uint32  VectorParamsAs1DForOutWhenUnconnected=off
  temp_state40 : Outport  Port=40  OutDataTypeStr=uint32  VectorParamsAs1DForOutWhenUnconnected=off
  temp_state41 : Outport  Port=41  OutDataTypeStr=uint32  VectorParamsAs1DForOutWhenUnconnected=off
  temp_state42 : Outport  Port=42  OutDataTypeStr=uint32  VectorParamsAs1DForOutWhenUnconnected=off
  temp_state43 : Outport  Port=43  OutDataTypeStr=uint32  VectorParamsAs1DForOutWhenUnconnected=off
  temp_state44 : Outport  Port=44  OutDataTypeStr=uint32  VectorParamsAs1DForOutWhenUnconnected=off
  complete : Outport  Port=45  OutDataTypeStr=boolean  VectorParamsAs1DForOutWhenUnconnected=off
  wires:
  Subsystem1/1(temp_state) -> temp_state3/1
  Subsystem5/1(temp_state) -> temp_state11/1
  Subsystem/2(temp_state1) -> temp_state2/1
  data2/1 -> Subsystem/3(data2)
  data1/1 -> Subsystem/2(data1)
  Subsystem1/2(temp_state1) -> temp_state4/1
  Subsystem/1(temp_state) -> temp_state1/1
  Subsystem6/1(temp_state) -> temp_state13/1
  Subsystem2/1(temp_state) -> temp_state5/1
  Subsystem2/2(temp_state1) -> temp_state6/1
  Subsystem3/1(temp_state) -> temp_state7/1
  Subsystem3/2(temp_state1) -> temp_state8/1
  Subsystem7/1(temp_state) -> temp_state15/1
  Subsystem5/2(temp_state1) -> temp_state12/1
  Subsystem7/2(temp_state1) -> temp_state16/1
  Subsystem6/2(temp_state1) -> temp_state14/1
  Subsystem4/1(temp_state) -> temp_state9/1
  Subsystem4/2(temp_state1) -> temp_state10/1
  Subsystem11/2(temp_state1) -> temp_state24/1
  Subsystem11/1(temp_state) -> temp_state23/1
  Subsystem9/1(temp_state) -> temp_state19/1
  Subsystem9/2(temp_state1) -> temp_state20/1
  Subsystem14/2(temp_state1) -> temp_state30/1
  Subsystem10/1(temp_state) -> temp_state21/1
  Subsystem14/1(temp_state) -> temp_state29/1
  Subsystem12/2(temp_state1) -> temp_state26/1
  Subsystem12/1(temp_state) -> temp_state25/1
  Subsystem13/1(temp_state) -> temp_state27/1
  Subsystem13/2(temp_state1) -> temp_state28/1
  Subsystem10/2(temp_state1) -> temp_state22/1
  Subsystem8/1(temp_state) -> temp_state17/1
  Subsystem8/2(temp_state1) -> temp_state18/1
  Subsystem15/1(temp_state) -> temp_state31/1
  Subsystem15/2(temp_state1) -> temp_state32/1
  Subsystem16/2(temp_state1) -> temp_state34/1
  Subsystem17/1(temp_state) -> temp_state35/1
  Subsystem18/2(temp_state1) -> temp_state38/1
  Subsystem17/2(temp_state1) -> temp_state36/1
  Subsystem18/1(temp_state) -> temp_state37/1
  Subsystem16/1(temp_state) -> temp_state33/1
  Subsystem19/1(temp_state) -> temp_state39/1
  Subsystem21/1(temp_state) -> temp_state43/1
  Subsystem20/2(temp_state1) -> temp_state42/1
  Subsystem21/2(temp_state1) -> temp_state44/1
  Subsystem20/1(temp_state) -> temp_state41/1
  Subsystem19/2(temp_state1) -> temp_state40/1
  data3/1 -> Subsystem1/2(data1)
  data4/1 -> Subsystem1/3(data2)
  data6/1 -> Subsystem2/3(data2)
  data7/1 -> Subsystem3/2(data1)
  data5/1 -> Subsystem2/2(data1)
  data8/1 -> Subsystem3/3(data2)
  data10/1 -> Subsystem4/3(data2)
  data13/1 -> Subsystem6/2(data1)
  data15/1 -> Subsystem7/2(data1)
  data14/1 -> Subsystem6/3(data2)
  data16/1 -> Subsystem7/3(data2)
  data11/1 -> Subsystem5/2(data1)
  data9/1 -> Subsystem4/2(data1)
  data12/1 -> Subsystem5/3(data2)
  data17/1 -> Subsystem8/2(data1)
  data18/1 -> Subsystem8/3(data2)
  data28/1 -> Subsystem13/3(data2)
  data25/1 -> Subsystem12/2(data1)
  data30/1 -> Subsystem14/3(data2)
  data21/1 -> Subsystem10/2(data1)
  data23/1 -> Subsystem11/2(data1)
  data27/1 -> Subsystem13/2(data1)
  data22/1 -> Subsystem10/3(data2)
  data24/1 -> Subsystem11/3(data2)
  data32/1 -> Subsystem15/3(data2)
  data31/1 -> Subsystem15/2(data1)
  data19/1 -> Subsystem9/2(data1)
  data26/1 -> Subsystem12/3(data2)
  data20/1 -> Subsystem9/3(data2)
  data29/1 -> Subsystem14/2(data1)
  data33/1 -> Subsystem16/2(data1)
  data34/1 -> Subsystem16/3(data2)
  data44/1 -> Subsystem21/3(data2)
  data41/1 -> Subsystem20/2(data1)
  data37/1 -> Subsystem18/2(data1)
  data39/1 -> Subsystem19/2(data1)
  data43/1 -> Subsystem21/2(data1)
  data38/1 -> Subsystem18/3(data2)
  data40/1 -> Subsystem19/3(data2)
  data35/1 -> Subsystem17/2(data1)
  data42/1 -> Subsystem20/3(data2)
  data36/1 -> Subsystem17/3(data2)
  we/1 -> Subsystem21/1(we), Subsystem20/1(we), Subsystem19/1(we), Subsystem18/1(we), Subsystem17/1(we), Subsystem16/1(we), Subsystem15/1(we), Subsystem14/1(we), Subsystem13/1(we), Subsystem12/1(we), Subsystem11/1(we), Subsystem10/1(we), Subsystem9/1(we), Subsystem8/1(we), Subsystem7/1(we), Subsystem6/1(we), Subsystem5/1(we), Subsystem4/1(we), Subsystem3/1(we), Subsystem2/1(we), Subsystem1/1(we), Subsystem/1(we), Delay/1
  Delay/1 -> complete/1

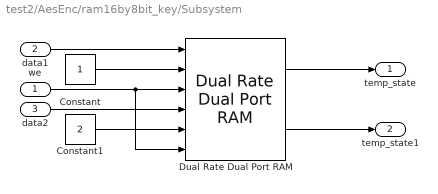
== system test2/AesEnc/ram16by8bit_key/Subsystem ==
  we : Inport  OutDataTypeStr=boolean
  data1 : Inport  Port=2  OutDataTypeStr=uint8
  data2 : Inport  Port=3  OutDataTypeStr=uint8
  Constant : Constant
  Constant1 : Constant  Value=2
  Dual Rate Dual Port RAM : hdlsllib/HDL RAMs/Dual Rate Dual Port RAM  ram_size=2
      settings: SourceProductBaseCode=SL
  temp_state : Outport  OutDataTypeStr=uint8  VectorParamsAs1DForOutWhenUnconnected=off
  temp_state1 : Outport  Port=2  OutDataTypeStr=uint8  VectorParamsAs1DForOutWhenUnconnected=off
  wires:
  Dual Rate Dual Port RAM/1 -> temp_state/1
  data2/1 -> Dual Rate Dual Port RAM/4
  Constant/1 -> Dual Rate Dual Port RAM/2
  data1/1 -> Dual Rate Dual Port RAM/1
  we/1 -> Dual Rate Dual Port RAM/6, Dual Rate Dual Port RAM/3
  Dual Rate Dual Port RAM/2 -> temp_state1/1
  Constant1/1 -> Dual Rate Dual Port RAM/5

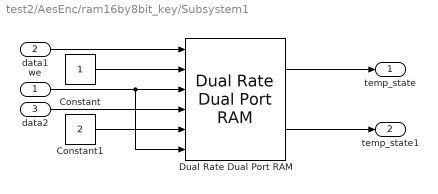
== system test2/AesEnc/ram16by8bit_key/Subsystem1 ==
  we : Inport  OutDataTypeStr=boolean
  data1 : Inport  Port=2  OutDataTypeStr=uint8
  data2 : Inport  Port=3  OutDataTypeStr=uint8
  Constant : Constant
  Constant1 : Constant  Value=2
  Dual Rate Dual Port RAM : hdlsllib/HDL RAMs/Dual Rate Dual Port RAM  ram_size=2
      settings: SourceProductBaseCode=SL
  temp_state : Outport  OutDataTypeStr=uint8  VectorParamsAs1DForOutWhenUnconnected=off
  temp_state1 : Outport  Port=2  OutDataTypeStr=uint8  VectorParamsAs1DForOutWhenUnconnected=off
  wires:
  Dual Rate Dual Port RAM/1 -> temp_state/1
  data2/1 -> Dual Rate Dual Port RAM/4
  Constant/1 -> Dual Rate Dual Port RAM/2
  data1/1 -> Dual Rate Dual Port RAM/1
  we/1 -> Dual Rate Dual Port RAM/6, Dual Rate Dual Port RAM/3
  Dual Rate Dual Port RAM/2 -> temp_state1/1
  Constant1/1 -> Dual Rate Dual Port RAM/5

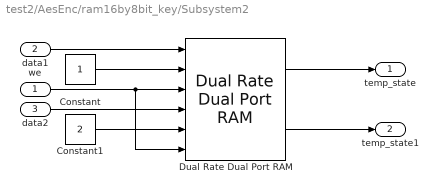
== system test2/AesEnc/ram16by8bit_key/Subsystem2 ==
  we : Inport  OutDataTypeStr=boolean
  data1 : Inport  Port=2  OutDataTypeStr=uint8
  data2 : Inport  Port=3  OutDataTypeStr=uint8
  Constant : Constant
  Constant1 : Constant  Value=2
  Dual Rate Dual Port RAM : hdlsllib/HDL RAMs/Dual Rate Dual Port RAM  ram_size=2
      settings: SourceProductBaseCode=SL
  temp_state : Outport  OutDataTypeStr=uint8  VectorParamsAs1DForOutWhenUnconnected=off
  temp_state1 : Outport  Port=2  OutDataTypeStr=uint8  VectorParamsAs1DForOutWhenUnconnected=off
  wires:
  Dual Rate Dual Port RAM/1 -> temp_state/1
  data2/1 -> Dual Rate Dual Port RAM/4
  Constant/1 -> Dual Rate Dual Port RAM/2
  data1/1 -> Dual Rate Dual Port RAM/1
  we/1 -> Dual Rate Dual Port RAM/6, Dual Rate Dual Port RAM/3
  Dual Rate Dual Port RAM/2 -> temp_state1/1
  Constant1/1 -> Dual Rate Dual Port RAM/5

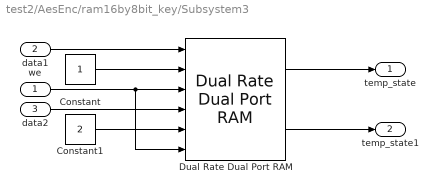
== system test2/AesEnc/ram16by8bit_key/Subsystem3 ==
  we : Inport  OutDataTypeStr=boolean
  data1 : Inport  Port=2  OutDataTypeStr=uint8
  data2 : Inport  Port=3  OutDataTypeStr=uint8
  Constant : Constant
  Constant1 : Constant  Value=2
  Dual Rate Dual Port RAM : hdlsllib/HDL RAMs/Dual Rate Dual Port RAM  ram_size=2
      settings: SourceProductBaseCode=SL
  temp_state : Outport  OutDataTypeStr=uint8  VectorParamsAs1DForOutWhenUnconnected=off
  temp_state1 : Outport  Port=2  OutDataTypeStr=uint8  VectorParamsAs1DForOutWhenUnconnected=off
  wires:
  Dual Rate Dual Port RAM/1 -> temp_state/1
  data2/1 -> Dual Rate Dual Port RAM/4
  Constant/1 -> Dual Rate Dual Port RAM/2
  data1/1 -> Dual Rate Dual Port RAM/1
  we/1 -> Dual Rate Dual Port RAM/6, Dual Rate Dual Port RAM/3
  Dual Rate Dual Port RAM/2 -> temp_state1/1
  Constant1/1 -> Dual Rate Dual Port RAM/5

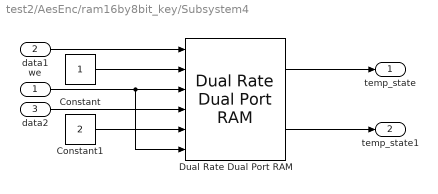
== system test2/AesEnc/ram16by8bit_key/Subsystem4 ==
  we : Inport  OutDataTypeStr=boolean
  data1 : Inport  Port=2  OutDataTypeStr=uint8
  data2 : Inport  Port=3  OutDataTypeStr=uint8
  Constant : Constant
  Constant1 : Constant  Value=2
  Dual Rate Dual Port RAM : hdlsllib/HDL RAMs/Dual Rate Dual Port RAM  ram_size=2
      settings: SourceProductBaseCode=SL
  temp_state : Outport  OutDataTypeStr=uint8  VectorParamsAs1DForOutWhenUnconnected=off
  temp_state1 : Outport  Port=2  OutDataTypeStr=uint8  VectorParamsAs1DForOutWhenUnconnected=off
  wires:
  Dual Rate Dual Port RAM/1 -> temp_state/1
  data2/1 -> Dual Rate Dual Port RAM/4
  Constant/1 -> Dual Rate Dual Port RAM/2
  data1/1 -> Dual Rate Dual Port RAM/1
  we/1 -> Dual Rate Dual Port RAM/6, Dual Rate Dual Port RAM/3
  Dual Rate Dual Port RAM/2 -> temp_state1/1
  Constant1/1 -> Dual Rate Dual Port RAM/5

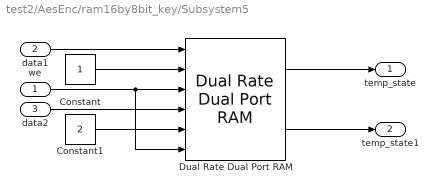
== system test2/AesEnc/ram16by8bit_key/Subsystem5 ==
  we : Inport  OutDataTypeStr=boolean
  data1 : Inport  Port=2  OutDataTypeStr=uint8
  data2 : Inport  Port=3  OutDataTypeStr=uint8
  Constant : Constant
  Constant1 : Constant  Value=2
  Dual Rate Dual Port RAM : hdlsllib/HDL RAMs/Dual Rate Dual Port RAM  ram_size=2
      settings: SourceProductBaseCode=SL
  temp_state : Outport  OutDataTypeStr=uint8  VectorParamsAs1DForOutWhenUnconnected=off
  temp_state1 : Outport  Port=2  OutDataTypeStr=uint8  VectorParamsAs1DForOutWhenUnconnected=off
  wires:
  Dual Rate Dual Port RAM/1 -> temp_state/1
  data2/1 -> Dual Rate Dual Port RAM/4
  Constant/1 -> Dual Rate Dual Port RAM/2
  data1/1 -> Dual Rate Dual Port RAM/1
  we/1 -> Dual Rate Dual Port RAM/6, Dual Rate Dual Port RAM/3
  Dual Rate Dual Port RAM/2 -> temp_state1/1
  Constant1/1 -> Dual Rate Dual Port RAM/5

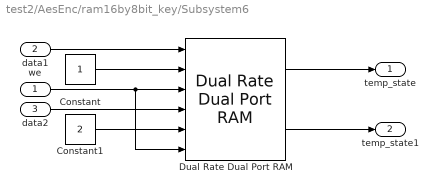
== system test2/AesEnc/ram16by8bit_key/Subsystem6 ==
  we : Inport  OutDataTypeStr=boolean
  data1 : Inport  Port=2  OutDataTypeStr=uint8
  data2 : Inport  Port=3  OutDataTypeStr=uint8
  Constant : Constant
  Constant1 : Constant  Value=2
  Dual Rate Dual Port RAM : hdlsllib/HDL RAMs/Dual Rate Dual Port RAM  ram_size=2
      settings: SourceProductBaseCode=SL
  temp_state : Outport  OutDataTypeStr=uint8  VectorParamsAs1DForOutWhenUnconnected=off
  temp_state1 : Outport  Port=2  OutDataTypeStr=uint8  VectorParamsAs1DForOutWhenUnconnected=off
  wires:
  Dual Rate Dual Port RAM/1 -> temp_state/1
  data2/1 -> Dual Rate Dual Port RAM/4
  Constant/1 -> Dual Rate Dual Port RAM/2
  data1/1 -> Dual Rate Dual Port RAM/1
  we/1 -> Dual Rate Dual Port RAM/6, Dual Rate Dual Port RAM/3
  Dual Rate Dual Port RAM/2 -> temp_state1/1
  Constant1/1 -> Dual Rate Dual Port RAM/5

== system test2/AesEnc/ram16by8bit_key/Subsystem7 ==
  we : Inport  OutDataTypeStr=boolean
  data1 : Inport  Port=2  OutDataTypeStr=uint8
  data2 : Inport  Port=3  OutDataTypeStr=uint8
  Constant : Constant
  Constant1 : Constant  Value=2
  Dual Rate Dual Port RAM : hdlsllib/HDL RAMs/Dual Rate Dual Port RAM  ram_size=2
      settings: SourceProductBaseCode=SL
  temp_state : Outport  OutDataTypeStr=uint8  VectorParamsAs1DForOutWhenUnconnected=off
  temp_state1 : Outport  Port=2  OutDataTypeStr=uint8  VectorParamsAs1DForOutWhenUnconnected=off
  wires:
  Dual Rate Dual Port RAM/1 -> temp_state/1
  data2/1 -> Dual Rate Dual Port RAM/4
  Constant/1 -> Dual Rate Dual Port RAM/2
  data1/1 -> Dual Rate Dual Port RAM/1
  we/1 -> Dual Rate Dual Port RAM/6, Dual Rate Dual Port RAM/3
  Dual Rate Dual Port RAM/2 -> temp_state1/1
  Constant1/1 -> Dual Rate Dual Port RAM/5

== system test2/AesEnc/ram16by8bit_state/Subsystem ==
  we : Inport  OutDataTypeStr=boolean
  data1 : Inport  Port=2  OutDataTypeStr=uint8
  data2 : Inport  Port=3  OutDataTypeStr=uint8
  Constant : Constant
  Constant1 : Constant  Value=2
  Dual Rate Dual Port RAM : hdlsllib/HDL RAMs/Dual Rate Dual Port RAM  ram_size=2
      settings: SourceProductBaseCode=SL
  temp_state : Outport  OutDataTypeStr=uint8  VectorParamsAs1DForOutWhenUnconnected=off
  temp_state1 : Outport  Port=2  OutDataTypeStr=uint8  VectorParamsAs1DForOutWhenUnconnected=off
  wires:
  Dual Rate Dual Port RAM/1 -> temp_state/1
  data2/1 -> Dual Rate Dual Port RAM/4
  Constant/1 -> Dual Rate Dual Port RAM/2
  data1/1 -> Dual Rate Dual Port RAM/1
  we/1 -> Dual Rate Dual Port RAM/6, Dual Rate Dual Port RAM/3
  Dual Rate Dual Port RAM/2 -> temp_state1/1
  Constant1/1 -> Dual Rate Dual Port RAM/5

== system test2/AesEnc/ram16by8bit_state/Subsystem1 ==
  we : Inport  OutDataTypeStr=boolean
  data1 : Inport  Port=2  OutDataTypeStr=uint8
  data2 : Inport  Port=3  OutDataTypeStr=uint8
  Constant : Constant
  Constant1 : Constant  Value=2
  Dual Rate Dual Port RAM : hdlsllib/HDL RAMs/Dual Rate Dual Port RAM  ram_size=2
      settings: SourceProductBaseCode=SL
  temp_state : Outport  OutDataTypeStr=uint8  VectorParamsAs1DForOutWhenUnconnected=off
  temp_state1 : Outport  Port=2  OutDataTypeStr=uint8  VectorParamsAs1DForOutWhenUnconnected=off
  wires:
  Dual Rate Dual Port RAM/1 -> temp_state/1
  data2/1 -> Dual Rate Dual Port RAM/4
  Constant/1 -> Dual Rate Dual Port RAM/2
  data1/1 -> Dual Rate Dual Port RAM/1
  we/1 -> Dual Rate Dual Port RAM/6, Dual Rate Dual Port RAM/3
  Dual Rate Dual Port RAM/2 -> temp_state1/1
  Constant1/1 -> Dual Rate Dual Port RAM/5

== system test2/AesEnc/ram16by8bit_state/Subsystem2 ==
  we : Inport  OutDataTypeStr=boolean
  data1 : Inport  Port=2  OutDataTypeStr=uint8
  data2 : Inport  Port=3  OutDataTypeStr=uint8
  Constant : Constant
  Constant1 : Constant  Value=2
  Dual Rate Dual Port RAM : hdlsllib/HDL RAMs/Dual Rate Dual Port RAM  ram_size=2
      settings: SourceProductBaseCode=SL
  temp_state : Outport  OutDataTypeStr=uint8  VectorParamsAs1DForOutWhenUnconnected=off
  temp_state1 : Outport  Port=2  OutDataTypeStr=uint8  VectorParamsAs1DForOutWhenUnconnected=off
  wires:
  Dual Rate Dual Port RAM/1 -> temp_state/1
  data2/1 -> Dual Rate Dual Port RAM/4
  Constant/1 -> Dual Rate Dual Port RAM/2
  data1/1 -> Dual Rate Dual Port RAM/1
  we/1 -> Dual Rate Dual Port RAM/6, Dual Rate Dual Port RAM/3
  Dual Rate Dual Port RAM/2 -> temp_state1/1
  Constant1/1 -> Dual Rate Dual Port RAM/5

== system test2/AesEnc/ram16by8bit_state/Subsystem3 ==
  we : Inport  OutDataTypeStr=boolean
  data1 : Inport  Port=2  OutDataTypeStr=uint8
  data2 : Inport  Port=3  OutDataTypeStr=uint8
  Constant : Constant
  Constant1 : Constant  Value=2
  Dual Rate Dual Port RAM : hdlsllib/HDL RAMs/Dual Rate Dual Port RAM  ram_size=2
      settings: SourceProductBaseCode=SL
  temp_state : Outport  OutDataTypeStr=uint8  VectorParamsAs1DForOutWhenUnconnected=off
  temp_state1 : Outport  Port=2  OutDataTypeStr=uint8  VectorParamsAs1DForOutWhenUnconnected=off
  wires:
  Dual Rate Dual Port RAM/1 -> temp_state/1
  data2/1 -> Dual Rate Dual Port RAM/4
  Constant/1 -> Dual Rate Dual Port RAM/2
  data1/1 -> Dual Rate Dual Port RAM/1
  we/1 -> Dual Rate Dual Port RAM/6, Dual Rate Dual Port RAM/3
  Dual Rate Dual Port RAM/2 -> temp_state1/1
  Constant1/1 -> Dual Rate Dual Port RAM/5

== system test2/AesEnc/ram16by8bit_state/Subsystem4 ==
  we : Inport  OutDataTypeStr=boolean
  data1 : Inport  Port=2  OutDataTypeStr=uint8
  data2 : Inport  Port=3  OutDataTypeStr=uint8
  Constant : Constant
  Constant1 : Constant  Value=2
  Dual Rate Dual Port RAM : hdlsllib/HDL RAMs/Dual Rate Dual Port RAM  ram_size=2
      settings: SourceProductBaseCode=SL
  temp_state : Outport  OutDataTypeStr=uint8  VectorParamsAs1DForOutWhenUnconnected=off
  temp_state1 : Outport  Port=2  OutDataTypeStr=uint8  VectorParamsAs1DForOutWhenUnconnected=off
  wires:
  Dual Rate Dual Port RAM/1 -> temp_state/1
  data2/1 -> Dual Rate Dual Port RAM/4
  Constant/1 -> Dual Rate Dual Port RAM/2
  data1/1 -> Dual Rate Dual Port RAM/1
  we/1 -> Dual Rate Dual Port RAM/6, Dual Rate Dual Port RAM/3
  Dual Rate Dual Port RAM/2 -> temp_state1/1
  Constant1/1 -> Dual Rate Dual Port RAM/5

== system test2/AesEnc/ram16by8bit_state/Subsystem5 ==
  we : Inport  OutDataTypeStr=boolean
  data1 : Inport  Port=2  OutDataTypeStr=uint8
  data2 : Inport  Port=3  OutDataTypeStr=uint8
  Constant : Constant
  Constant1 : Constant  Value=2
  Dual Rate Dual Port RAM : hdlsllib/HDL RAMs/Dual Rate Dual Port RAM  ram_size=2
      settings: SourceProductBaseCode=SL
  temp_state : Outport  OutDataTypeStr=uint8  VectorParamsAs1DForOutWhenUnconnected=off
  temp_state1 : Outport  Port=2  OutDataTypeStr=uint8  VectorParamsAs1DForOutWhenUnconnected=off
  wires:
  Dual Rate Dual Port RAM/1 -> temp_state/1
  data2/1 -> Dual Rate Dual Port RAM/4
  Constant/1 -> Dual Rate Dual Port RAM/2
  data1/1 -> Dual Rate Dual Port RAM/1
  we/1 -> Dual Rate Dual Port RAM/6, Dual Rate Dual Port RAM/3
  Dual Rate Dual Port RAM/2 -> temp_state1/1
  Constant1/1 -> Dual Rate Dual Port RAM/5

== system test2/AesEnc/ram16by8bit_state/Subsystem6 ==
  we : Inport  OutDataTypeStr=boolean
  data1 : Inport  Port=2  OutDataTypeStr=uint8
  data2 : Inport  Port=3  OutDataTypeStr=uint8
  Constant : Constant
  Constant1 : Constant  Value=2
  Dual Rate Dual Port RAM : hdlsllib/HDL RAMs/Dual Rate Dual Port RAM  ram_size=2
      settings: SourceProductBaseCode=SL
  temp_state : Outport  OutDataTypeStr=uint8  VectorParamsAs1DForOutWhenUnconnected=off
  temp_state1 : Outport  Port=2  OutDataTypeStr=uint8  VectorParamsAs1DForOutWhenUnconnected=off
  wires:
  Dual Rate Dual Port RAM/1 -> temp_state/1
  data2/1 -> Dual Rate Dual Port RAM/4
  Constant/1 -> Dual Rate Dual Port RAM/2
  data1/1 -> Dual Rate Dual Port RAM/1
  we/1 -> Dual Rate Dual Port RAM/6, Dual Rate Dual Port RAM/3
  Dual Rate Dual Port RAM/2 -> temp_state1/1
  Constant1/1 -> Dual Rate Dual Port RAM/5

== system test2/AesEnc/ram16by8bit_state/Subsystem7 ==
  we : Inport  OutDataTypeStr=boolean
  data1 : Inport  Port=2  OutDataTypeStr=uint8
  data2 : Inport  Port=3  OutDataTypeStr=uint8
  Constant : Constant
  Constant1 : Constant  Value=2
  Dual Rate Dual Port RAM : hdlsllib/HDL RAMs/Dual Rate Dual Port RAM  ram_size=2
      settings: SourceProductBaseCode=SL
  temp_state : Outport  OutDataTypeStr=uint8  VectorParamsAs1DForOutWhenUnconnected=off
  temp_state1 : Outport  Port=2  OutDataTypeStr=uint8  VectorParamsAs1DForOutWhenUnconnected=off
  wires:
  Dual Rate Dual Port RAM/1 -> temp_state/1
  data2/1 -> Dual Rate Dual Port RAM/4
  Constant/1 -> Dual Rate Dual Port RAM/2
  data1/1 -> Dual Rate Dual Port RAM/1
  we/1 -> Dual Rate Dual Port RAM/6, Dual Rate Dual Port RAM/3
  Dual Rate Dual Port RAM/2 -> temp_state1/1
  Constant1/1 -> Dual Rate Dual Port RAM/5
